simulink model "MultipleCoordinator"  (R2021b)
settings: Solver=FixedStepDiscrete  StartTime=0.0  StopTime=10.0  RelTol=1e-3
undefined symbols (not defined in the file): sldvsubsys
libraries: simulink x8, sldvlib x4
settings Model: Creator=Alessandro  LastModifiedBy=Mattia
settings ConfigComp: DVMode=PropertyProving  DVTestSuiteOptimization=Auto  DVDetectOutOfBounds=on  DVModelReferenceHarness=on

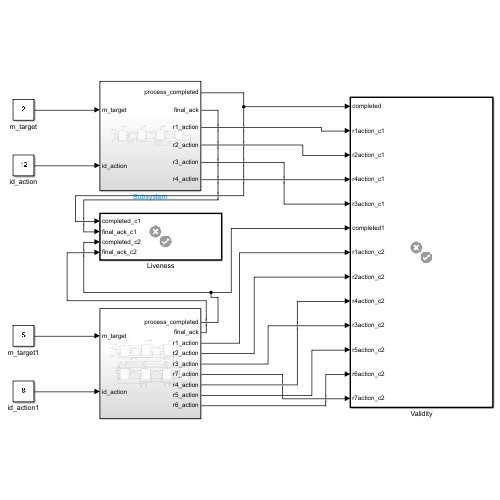
[thumbnail: Simulink's stored preview of the top-level diagram]
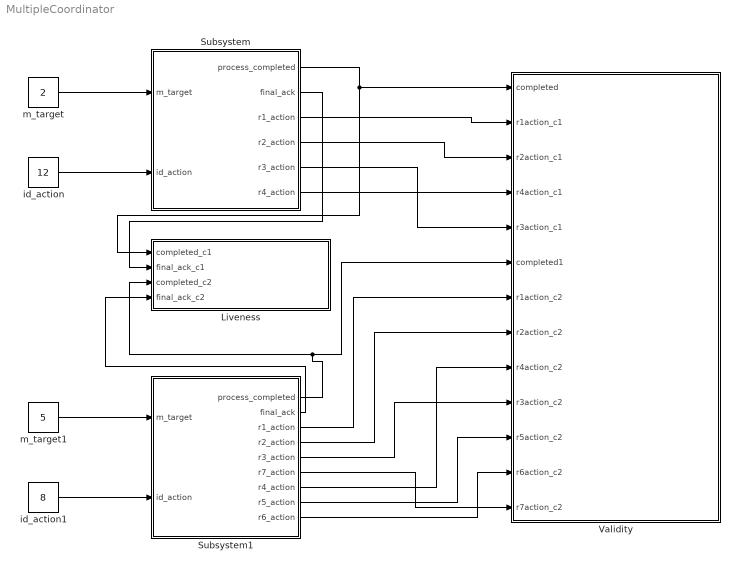
== system MultipleCoordinator ==
  Liveness : Subsystem  Tag=VerificationSubsystem  DisableCoverage=on  LoadFcn=sldvsubsys('check')  TreatAsAtomicUnit=on  SimViewingDevice=on  mask(VerificationSubsystem){}
      mask init:
      | sldvsubsys('maskInit');
      settings: CopyFcn=sldvsubsys('copy');  OpenFcn=open_system(gcb,'force');
      settings: PreSaveFcn=|
      | set_param(gcb,'SimViewingDevice','on');
      | sldvsubsys('check');
      mask Help: helpview(fullfile(docroot,'toolbox','sldv','sldv.map'),'verificationsubsystem')
      mask Display: image(imread('sldvicon_versubsys.png','BackGroundColor',[1 1 1]),'center');
  Subsystem : Subsystem
  Subsystem1 : Subsystem
  Validity : Subsystem  Tag=VerificationSubsystem  DisableCoverage=on  LoadFcn=sldvsubsys('check')  TreatAsAtomicUnit=on  SimViewingDevice=on  mask(VerificationSubsystem){}
      mask init:
      | sldvsubsys('maskInit');
      settings: CopyFcn=sldvsubsys('copy');  OpenFcn=open_system(gcb,'force');
      settings: PreSaveFcn=|
      | set_param(gcb,'SimViewingDevice','on');
      | sldvsubsys('check');
      mask Help: helpview(fullfile(docroot,'toolbox','sldv','sldv.map'),'verificationsubsystem')
      mask Display: image(imread('sldvicon_versubsys.png','BackGroundColor',[1 1 1]),'center');
  id_action : Constant  Value=12
  id_action1 : Constant  Value=8
  m_target : Constant  Value=2
  m_target1 : Constant  Value=5
  wires:
  m_target/1 -> Subsystem/1(m_target)
  id_action/1 -> Subsystem/2(id_action)
  Subsystem/1(process_completed) -> Liveness/1(completed_c1), Validity/1(completed)
  Subsystem/2(final_ack) -> Liveness/2(final_ack_c1)
  Subsystem/3(r1_action) -> Validity/2(r1action_c1)
  Subsystem/4(r2_action) -> Validity/3(r2action_c1)
  Subsystem/5(r3_action) -> Validity/5(r3action_c1)
  Subsystem/6(r4_action) -> Validity/4(r4action_c1)
  Subsystem1/2(final_ack) -> Liveness/4(final_ack_c2)
  id_action1/1 -> Subsystem1/2(id_action)
  m_target1/1 -> Subsystem1/1(m_target)
  Subsystem1/1(process_completed) -> Validity/6(completed1), Liveness/3(completed_c2)
  Subsystem1/3(r1_action) -> Validity/7(r1action_c2)
  Subsystem1/4(r2_action) -> Validity/8(r2action_c2)
  Subsystem1/7(r4_action) -> Validity/9(r4action_c2)
  Subsystem1/5(r3_action) -> Validity/10(r3action_c2)
  Subsystem1/8(r5_action) -> Validity/11(r5action_c2)
  Subsystem1/9(r6_action) -> Validity/12(r6action_c2)
  Subsystem1/6(r7_action) -> Validity/13(r7action_c2)

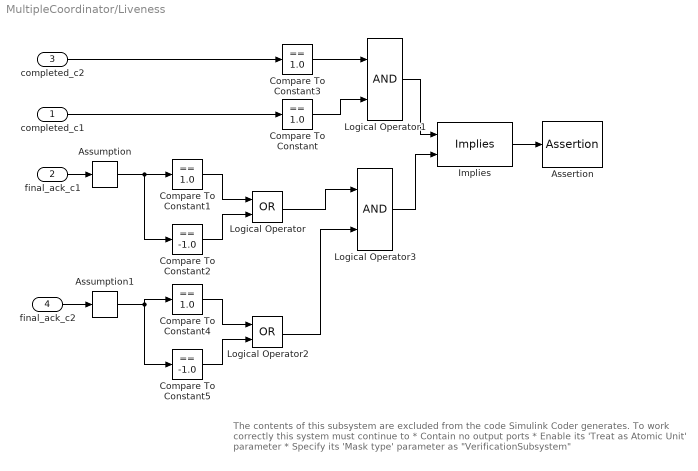
== system MultipleCoordinator/Liveness ==
  note: The contents of this subsystem are excluded from the code Simulink Coder
      | generates.
      |
      | To work correctly this system must continue to
      | * Contain no output ports
      | * Enable its 'Treat as Atomic Unit' parameter
      | * Specify its 'Mask type' parameter as "VerificationSubsystem"
  completed_c1 : Inport
  final_ack_c1 : Inport  Port=2
  completed_c2 : Inport  Port=3
  final_ack_c2 : Inport  Port=4
  Assertion : Assertion
  Assumption : sldvlib/Objectives and Constraints/Assumption  enabled=off  customAVTBlockType=Assumption  intervals={-1,1}  initial=off  dispValues=on  outEnabled=on
      settings: AttributesFormatString=%<intervals>  SourceProductBaseCode=SL
  Assumption1 : sldvlib/Objectives and Constraints/Assumption  enabled=off  customAVTBlockType=Assumption  intervals={-1,1}  initial=off  dispValues=on  outEnabled=on
      settings: AttributesFormatString=%<intervals>  SourceProductBaseCode=SL
  Compare To Constant{,1,3..4} (4 alike) : simulink/Logic and Bit Operations/Compare To Constant  relop===  const=1.0  OutDataTypeStr=boolean
  Compare To Constant2 : simulink/Logic and Bit Operations/Compare To Constant  relop===  const=-1.0  OutDataTypeStr=boolean
  Compare To Constant5 : simulink/Logic and Bit Operations/Compare To Constant  relop===  const=-1.0  OutDataTypeStr=boolean
  Implies : sldvlib/Verification Utilities/Implies
      settings: SourceProductBaseCode=SL
  Logical Operator : Logic  Operator=OR  AllPortsSameDT=off  OutDataTypeStr=boolean
  Logical Operator1 : Logic  AllPortsSameDT=off  OutDataTypeStr=boolean
  Logical Operator2 : Logic  Operator=OR  AllPortsSameDT=off  OutDataTypeStr=boolean
  Logical Operator3 : Logic  AllPortsSameDT=off  OutDataTypeStr=boolean
  wires:
  completed_c1/1 -> Compare To Constant/1
  Compare To Constant1/1 -> Logical Operator/1
  Compare To Constant2/1 -> Logical Operator/2
  Implies/1 -> Assertion/1
  final_ack_c1/1 -> Assumption/1
  Assumption/1 -> Compare To Constant2/1, Compare To Constant1/1
  completed_c2/1 -> Compare To Constant3/1
  Compare To Constant3/1 -> Logical Operator1/1
  Compare To Constant/1 -> Logical Operator1/2
  Compare To Constant4/1 -> Logical Operator2/1
  Compare To Constant5/1 -> Logical Operator2/2
  final_ack_c2/1 -> Assumption1/1
  Logical Operator1/1 -> Implies/1
  Logical Operator/1 -> Logical Operator3/1
  Logical Operator2/1 -> Logical Operator3/2
  Logical Operator3/1 -> Implies/2
  Assumption1/1 -> Compare To Constant4/1, Compare To Constant5/1

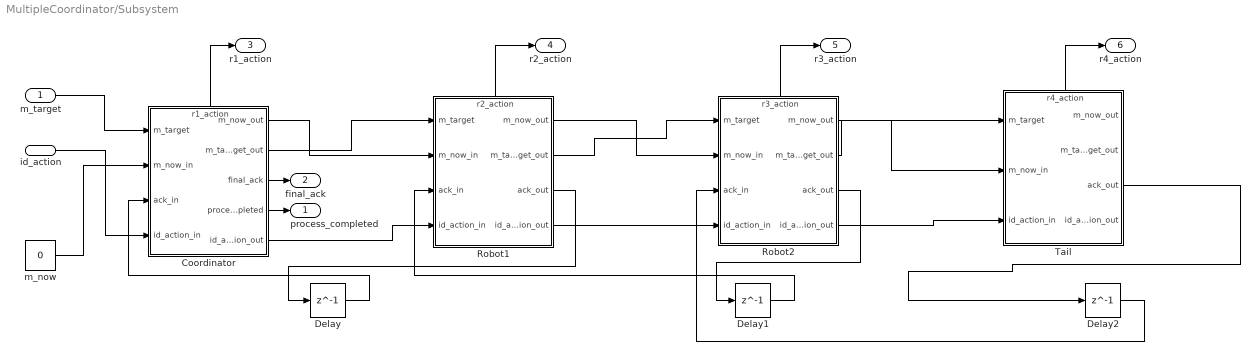
== system MultipleCoordinator/Subsystem ==
  m_target : Inport
  id_action : Inport  Port=2
  Coordinator : Stateflow chart  TreatAsAtomicUnit=on
      settings: PortSchema="{\"entries\":[{\"content\":{\"sides\":[{\"content\":{\"connectorIds\":[\"In1\",\"In2\",\"In3\",\"In4\"]},\"type\":\"ConnectorPlacement.EquallySpacedRectSide\",\"uuid\":\"f207236c-0599-4b46-9b3f-c0f809d9e1de\"},{\"content\":{\"connectorIds\":[\"Out2\",\"Out3\",\"Out4\",\"Out5\",\"Out6\"],\"side\":\"RIGHT\"},\"type\":\"ConnectorPlacement.EquallySpacedRectSide\",\"uuid\":\"63272974-e9ab-41b4-a3ca-cff66dd5b970\"},{\"content\":{\"connectorIds\":[\"Out1\"],\"side\":\"TOP\"},\"type\":\"ConnectorPlacement.EquallySpacedRectSide\",\"uuid\":\"6ce3df78-5d10-4d9a-bb6f-21eee9393606\"}]},\"type\":\"ConnectorPlacement.EquallySpacedConnector\",\"uuid\":\"1a0d068b-3bbf-4b25-a405-60ce12d31816\"}],\"packageUris\":[\"http://schema.mathworks.com/mf0/Connector/R2020b\"],\"version\":\"1.0\"}"
  Delay : Delay  DelayLength=1  InitialCondition=0
  Delay1 : Delay  DelayLength=1  InitialCondition=0
  Delay2 : Delay  DelayLength=1  InitialCondition=0
  Robot1 : Stateflow chart  TreatAsAtomicUnit=on
      settings: PortSchema="{\"entries\":[{\"content\":{\"sides\":[{\"content\":{\"connectorIds\":[\"In1\",\"In2\",\"In3\",\"In4\"]},\"type\":\"ConnectorPlacement.EquallySpacedRectSide\",\"uuid\":\"0bb30c5a-43df-4072-a77c-4a1dce14f9fe\"},{\"content\":{\"connectorIds\":[\"Out2\",\"Out3\",\"Out4\",\"Out5\"],\"side\":\"RIGHT\"},\"type\":\"ConnectorPlacement.EquallySpacedRectSide\",\"uuid\":\"e534c186-56c2-4af4-b3f1-02d020398bac\"},{\"content\":{\"connectorIds\":[\"Out1\"],\"side\":\"TOP\"},\"type\":\"ConnectorPlacement.EquallySpacedRectSide\",\"uuid\":\"e2ef603c-6980-4fc1-bc1c-88b0ffffdb44\"}]},\"type\":\"ConnectorPlacement.EquallySpacedConnector\",\"uuid\":\"7e88c6c9-7de7-4b98-93fa-510699497ff0\"}],\"packageUris\":[\"http://schema.mathworks.com/mf0/Connector/R2020b\"],\"version\":\"1.0\"}"
  Robot2 : Stateflow chart  TreatAsAtomicUnit=on
      settings: PortSchema="{\"entries\":[{\"content\":{\"sides\":[{\"content\":{\"connectorIds\":[\"In1\",\"In2\",\"In3\",\"In4\"]},\"type\":\"ConnectorPlacement.EquallySpacedRectSide\",\"uuid\":\"0bb30c5a-43df-4072-a77c-4a1dce14f9fe\"},{\"content\":{\"connectorIds\":[\"Out2\",\"Out3\",\"Out4\",\"Out5\"],\"side\":\"RIGHT\"},\"type\":\"ConnectorPlacement.EquallySpacedRectSide\",\"uuid\":\"e534c186-56c2-4af4-b3f1-02d020398bac\"},{\"content\":{\"connectorIds\":[\"Out1\"],\"side\":\"TOP\"},\"type\":\"ConnectorPlacement.EquallySpacedRectSide\",\"uuid\":\"e2ef603c-6980-4fc1-bc1c-88b0ffffdb44\"}]},\"type\":\"ConnectorPlacement.EquallySpacedConnector\",\"uuid\":\"7e88c6c9-7de7-4b98-93fa-510699497ff0\"}],\"packageUris\":[\"http://schema.mathworks.com/mf0/Connector/R2020b\"],\"version\":\"1.0\"}"
  Tail : Stateflow chart  TreatAsAtomicUnit=on
      settings: PortSchema="{\"entries\":[{\"content\":{\"sides\":[{\"content\":{\"connectorIds\":[\"In1\",\"In2\",\"In3\"]},\"type\":\"ConnectorPlacement.EquallySpacedRectSide\",\"uuid\":\"8f0c7a78-6297-425d-9fc8-91e71c821e74\"},{\"content\":{\"connectorIds\":[\"Out2\",\"Out3\",\"Out4\",\"Out5\"],\"side\":\"RIGHT\"},\"type\":\"ConnectorPlacement.EquallySpacedRectSide\",\"uuid\":\"2a4e4ba2-0ea2-4b66-9720-65f8c6802208\"},{\"content\":{\"connectorIds\":[\"Out1\"],\"side\":\"TOP\"},\"type\":\"ConnectorPlacement.EquallySpacedRectSide\",\"uuid\":\"3c4e4337-d1ab-4209-abe4-e09ccc9a45b1\"}]},\"type\":\"ConnectorPlacement.EquallySpacedConnector\",\"uuid\":\"5f75d573-6dad-4549-ba0d-242a5d54a9e5\"}],\"packageUris\":[\"http://schema.mathworks.com/mf0/Connector/R2020b\"],\"version\":\"1.0\"}"
  m_now : Constant  Value=0
  process_completed : Outport
  final_ack : Outport  Port=2
  r1_action : Outport  Port=3
  r2_action : Outport  Port=4
  r3_action : Outport  Port=5
  r4_action : Outport  Port=6
  wires:
  m_now/1 -> Coordinator/2(m_now_in)
  m_target/1 -> Coordinator/1(m_target)
  Delay/1 -> Coordinator/3(ack_in)
  Coordinator/2(m_now_out) -> Robot1/2(m_now_in)
  Coordinator/3(m_target_out) -> Robot1/1(m_target)
  Robot1/4(ack_out) -> Delay/1
  Coordinator/5(process_completed) -> process_completed/1
  Coordinator/4(final_ack) -> final_ack/1
  id_action/1 -> Coordinator/4(id_action_in)
  Coordinator/6(id_action_out) -> Robot1/4(id_action_in)
  Robot1/2(m_now_out) -> Robot2/2(m_now_in)
  Robot1/3(m_target_out) -> Robot2/1(m_target)
  Robot1/5(id_action_out) -> Robot2/4(id_action_in)
  Robot2/2(m_now_out) -> Tail/2(m_now_in)
  Robot2/3(m_target_out) -> Tail/1(m_target)
  Robot2/5(id_action_out) -> Tail/3(id_action_in)
  Robot2/4(ack_out) -> Delay1/1
  Delay1/1 -> Robot1/3(ack_in)
  Tail/4(ack_out) -> Delay2/1
  Delay2/1 -> Robot2/3(ack_in)
  Coordinator/1(r1_action) -> r1_action/1
  Robot1/1(r2_action) -> r2_action/1
  Robot2/1(r3_action) -> r3_action/1
  Tail/1(r4_action) -> r4_action/1

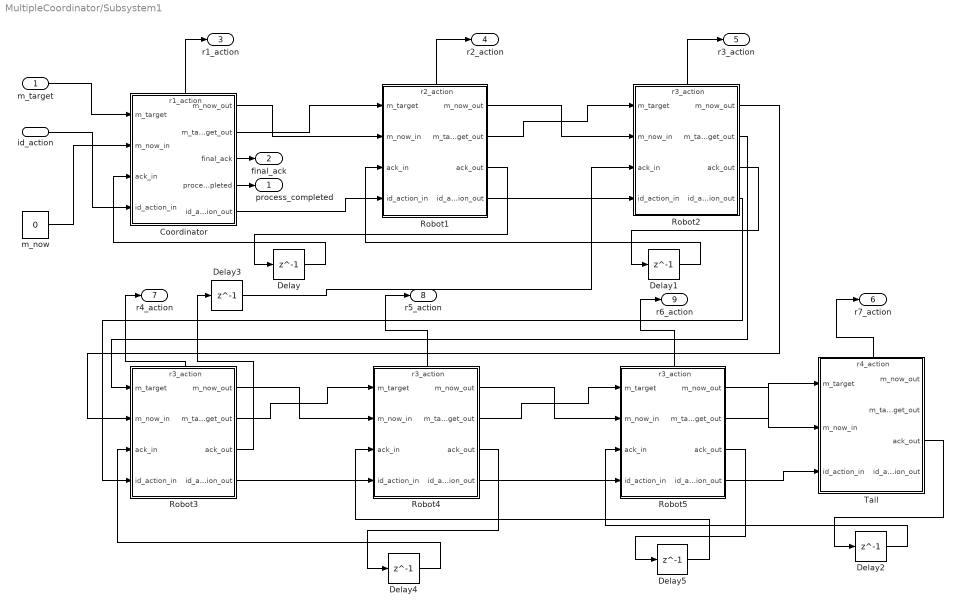
== system MultipleCoordinator/Subsystem1 ==
  m_target : Inport
  id_action : Inport  Port=2
  Coordinator : Stateflow chart  TreatAsAtomicUnit=on
      settings: PortSchema="{\"entries\":[{\"content\":{\"sides\":[{\"content\":{\"connectorIds\":[\"In1\",\"In2\",\"In3\",\"In4\"]},\"type\":\"ConnectorPlacement.EquallySpacedRectSide\",\"uuid\":\"f207236c-0599-4b46-9b3f-c0f809d9e1de\"},{\"content\":{\"connectorIds\":[\"Out2\",\"Out3\",\"Out4\",\"Out5\",\"Out6\"],\"side\":\"RIGHT\"},\"type\":\"ConnectorPlacement.EquallySpacedRectSide\",\"uuid\":\"63272974-e9ab-41b4-a3ca-cff66dd5b970\"},{\"content\":{\"connectorIds\":[\"Out1\"],\"side\":\"TOP\"},\"type\":\"ConnectorPlacement.EquallySpacedRectSide\",\"uuid\":\"6ce3df78-5d10-4d9a-bb6f-21eee9393606\"}]},\"type\":\"ConnectorPlacement.EquallySpacedConnector\",\"uuid\":\"1a0d068b-3bbf-4b25-a405-60ce12d31816\"}],\"packageUris\":[\"http://schema.mathworks.com/mf0/Connector/R2020b\"],\"version\":\"1.0\"}"
  Delay{,1..5} (6 alike) : Delay  DelayLength=1  InitialCondition=0
  Robot1 : Stateflow chart  TreatAsAtomicUnit=on
      settings: PortSchema="{\"entries\":[{\"content\":{\"sides\":[{\"content\":{\"connectorIds\":[\"In1\",\"In2\",\"In3\",\"In4\"]},\"type\":\"ConnectorPlacement.EquallySpacedRectSide\",\"uuid\":\"0bb30c5a-43df-4072-a77c-4a1dce14f9fe\"},{\"content\":{\"connectorIds\":[\"Out2\",\"Out3\",\"Out4\",\"Out5\"],\"side\":\"RIGHT\"},\"type\":\"ConnectorPlacement.EquallySpacedRectSide\",\"uuid\":\"e534c186-56c2-4af4-b3f1-02d020398bac\"},{\"content\":{\"connectorIds\":[\"Out1\"],\"side\":\"TOP\"},\"type\":\"ConnectorPlacement.EquallySpacedRectSide\",\"uuid\":\"e2ef603c-6980-4fc1-bc1c-88b0ffffdb44\"}]},\"type\":\"ConnectorPlacement.EquallySpacedConnector\",\"uuid\":\"7e88c6c9-7de7-4b98-93fa-510699497ff0\"}],\"packageUris\":[\"http://schema.mathworks.com/mf0/Connector/R2020b\"],\"version\":\"1.0\"}"
  Robot2 : Stateflow chart  TreatAsAtomicUnit=on
      settings: PortSchema="{\"entries\":[{\"content\":{\"sides\":[{\"content\":{\"connectorIds\":[\"In1\",\"In2\",\"In3\",\"In4\"]},\"type\":\"ConnectorPlacement.EquallySpacedRectSide\",\"uuid\":\"0bb30c5a-43df-4072-a77c-4a1dce14f9fe\"},{\"content\":{\"connectorIds\":[\"Out2\",\"Out3\",\"Out4\",\"Out5\"],\"side\":\"RIGHT\"},\"type\":\"ConnectorPlacement.EquallySpacedRectSide\",\"uuid\":\"e534c186-56c2-4af4-b3f1-02d020398bac\"},{\"content\":{\"connectorIds\":[\"Out1\"],\"side\":\"TOP\"},\"type\":\"ConnectorPlacement.EquallySpacedRectSide\",\"uuid\":\"e2ef603c-6980-4fc1-bc1c-88b0ffffdb44\"}]},\"type\":\"ConnectorPlacement.EquallySpacedConnector\",\"uuid\":\"7e88c6c9-7de7-4b98-93fa-510699497ff0\"}],\"packageUris\":[\"http://schema.mathworks.com/mf0/Connector/R2020b\"],\"version\":\"1.0\"}"
  Robot3 : Stateflow chart  TreatAsAtomicUnit=on
      settings: PortSchema="{\"entries\":[{\"content\":{\"sides\":[{\"content\":{\"connectorIds\":[\"In1\",\"In2\",\"In3\",\"In4\"]},\"type\":\"ConnectorPlacement.EquallySpacedRectSide\",\"uuid\":\"0bb30c5a-43df-4072-a77c-4a1dce14f9fe\"},{\"content\":{\"connectorIds\":[\"Out2\",\"Out3\",\"Out4\",\"Out5\"],\"side\":\"RIGHT\"},\"type\":\"ConnectorPlacement.EquallySpacedRectSide\",\"uuid\":\"e534c186-56c2-4af4-b3f1-02d020398bac\"},{\"content\":{\"connectorIds\":[\"Out1\"],\"side\":\"TOP\"},\"type\":\"ConnectorPlacement.EquallySpacedRectSide\",\"uuid\":\"e2ef603c-6980-4fc1-bc1c-88b0ffffdb44\"}]},\"type\":\"ConnectorPlacement.EquallySpacedConnector\",\"uuid\":\"7e88c6c9-7de7-4b98-93fa-510699497ff0\"}],\"packageUris\":[\"http://schema.mathworks.com/mf0/Connector/R2020b\"],\"version\":\"1.0\"}"
  Robot4 : Stateflow chart  TreatAsAtomicUnit=on
      settings: PortSchema="{\"entries\":[{\"content\":{\"sides\":[{\"content\":{\"connectorIds\":[\"In1\",\"In2\",\"In3\",\"In4\"]},\"type\":\"ConnectorPlacement.EquallySpacedRectSide\",\"uuid\":\"0bb30c5a-43df-4072-a77c-4a1dce14f9fe\"},{\"content\":{\"connectorIds\":[\"Out2\",\"Out3\",\"Out4\",\"Out5\"],\"side\":\"RIGHT\"},\"type\":\"ConnectorPlacement.EquallySpacedRectSide\",\"uuid\":\"e534c186-56c2-4af4-b3f1-02d020398bac\"},{\"content\":{\"connectorIds\":[\"Out1\"],\"side\":\"TOP\"},\"type\":\"ConnectorPlacement.EquallySpacedRectSide\",\"uuid\":\"e2ef603c-6980-4fc1-bc1c-88b0ffffdb44\"}]},\"type\":\"ConnectorPlacement.EquallySpacedConnector\",\"uuid\":\"7e88c6c9-7de7-4b98-93fa-510699497ff0\"}],\"packageUris\":[\"http://schema.mathworks.com/mf0/Connector/R2020b\"],\"version\":\"1.0\"}"
  Robot5 : Stateflow chart  TreatAsAtomicUnit=on
      settings: PortSchema="{\"entries\":[{\"content\":{\"sides\":[{\"content\":{\"connectorIds\":[\"In1\",\"In2\",\"In3\",\"In4\"]},\"type\":\"ConnectorPlacement.EquallySpacedRectSide\",\"uuid\":\"0bb30c5a-43df-4072-a77c-4a1dce14f9fe\"},{\"content\":{\"connectorIds\":[\"Out2\",\"Out3\",\"Out4\",\"Out5\"],\"side\":\"RIGHT\"},\"type\":\"ConnectorPlacement.EquallySpacedRectSide\",\"uuid\":\"e534c186-56c2-4af4-b3f1-02d020398bac\"},{\"content\":{\"connectorIds\":[\"Out1\"],\"side\":\"TOP\"},\"type\":\"ConnectorPlacement.EquallySpacedRectSide\",\"uuid\":\"e2ef603c-6980-4fc1-bc1c-88b0ffffdb44\"}]},\"type\":\"ConnectorPlacement.EquallySpacedConnector\",\"uuid\":\"7e88c6c9-7de7-4b98-93fa-510699497ff0\"}],\"packageUris\":[\"http://schema.mathworks.com/mf0/Connector/R2020b\"],\"version\":\"1.0\"}"
  Tail : Stateflow chart  TreatAsAtomicUnit=on
      settings: PortSchema="{\"entries\":[{\"content\":{\"sides\":[{\"content\":{\"connectorIds\":[\"In1\",\"In2\",\"In3\"]},\"type\":\"ConnectorPlacement.EquallySpacedRectSide\",\"uuid\":\"8f0c7a78-6297-425d-9fc8-91e71c821e74\"},{\"content\":{\"connectorIds\":[\"Out2\",\"Out3\",\"Out4\",\"Out5\"],\"side\":\"RIGHT\"},\"type\":\"ConnectorPlacement.EquallySpacedRectSide\",\"uuid\":\"2a4e4ba2-0ea2-4b66-9720-65f8c6802208\"},{\"content\":{\"connectorIds\":[\"Out1\"],\"side\":\"TOP\"},\"type\":\"ConnectorPlacement.EquallySpacedRectSide\",\"uuid\":\"3c4e4337-d1ab-4209-abe4-e09ccc9a45b1\"}]},\"type\":\"ConnectorPlacement.EquallySpacedConnector\",\"uuid\":\"5f75d573-6dad-4549-ba0d-242a5d54a9e5\"}],\"packageUris\":[\"http://schema.mathworks.com/mf0/Connector/R2020b\"],\"version\":\"1.0\"}"
  m_now : Constant  Value=0
  process_completed : Outport
  final_ack : Outport  Port=2
  r1_action : Outport  Port=3
  r2_action : Outport  Port=4
  r3_action : Outport  Port=5
  r7_action : Outport  Port=6
  r4_action : Outport  Port=7
  r5_action : Outport  Port=8
  r6_action : Outport  Port=9
  wires:
  m_now/1 -> Coordinator/2(m_now_in)
  m_target/1 -> Coordinator/1(m_target)
  Delay/1 -> Coordinator/3(ack_in)
  Coordinator/2(m_now_out) -> Robot1/2(m_now_in)
  Coordinator/3(m_target_out) -> Robot1/1(m_target)
  Robot1/4(ack_out) -> Delay/1
  Coordinator/5(process_completed) -> process_completed/1
  Coordinator/4(final_ack) -> final_ack/1
  id_action/1 -> Coordinator/4(id_action_in)
  Coordinator/6(id_action_out) -> Robot1/4(id_action_in)
  Robot1/2(m_now_out) -> Robot2/2(m_now_in)
  Robot1/3(m_target_out) -> Robot2/1(m_target)
  Robot1/5(id_action_out) -> Robot2/4(id_action_in)
  Robot2/4(ack_out) -> Delay1/1
  Delay1/1 -> Robot1/3(ack_in)
  Tail/4(ack_out) -> Delay2/1
  Coordinator/1(r1_action) -> r1_action/1
  Robot1/1(r2_action) -> r2_action/1
  Robot2/1(r3_action) -> r3_action/1
  Tail/1(r4_action) -> r7_action/1
  Robot2/3(m_target_out) -> Robot3/1(m_target)
  Robot3/1(r3_action) -> r4_action/1
  Delay3/1 -> Robot2/3(ack_in)
  Robot3/4(ack_out) -> Delay3/1
  Robot2/5(id_action_out) -> Robot3/4(id_action_in)
  Robot2/2(m_now_out) -> Robot3/2(m_now_in)
  Robot3/3(m_target_out) -> Robot4/1(m_target)
  Robot4/1(r3_action) -> r5_action/1
  Delay4/1 -> Robot3/3(ack_in)
  Robot4/4(ack_out) -> Delay4/1
  Robot3/5(id_action_out) -> Robot4/4(id_action_in)
  Robot3/2(m_now_out) -> Robot4/2(m_now_in)
  Robot4/3(m_target_out) -> Robot5/1(m_target)
  Robot5/1(r3_action) -> r6_action/1
  Delay5/1 -> Robot4/3(ack_in)
  Robot5/4(ack_out) -> Delay5/1
  Robot4/5(id_action_out) -> Robot5/4(id_action_in)
  Robot4/2(m_now_out) -> Robot5/2(m_now_in)
  Robot5/3(m_target_out) -> Tail/1(m_target)
  Robot5/2(m_now_out) -> Tail/2(m_now_in)
  Delay2/1 -> Robot5/3(ack_in)
  Robot5/5(id_action_out) -> Tail/3(id_action_in)

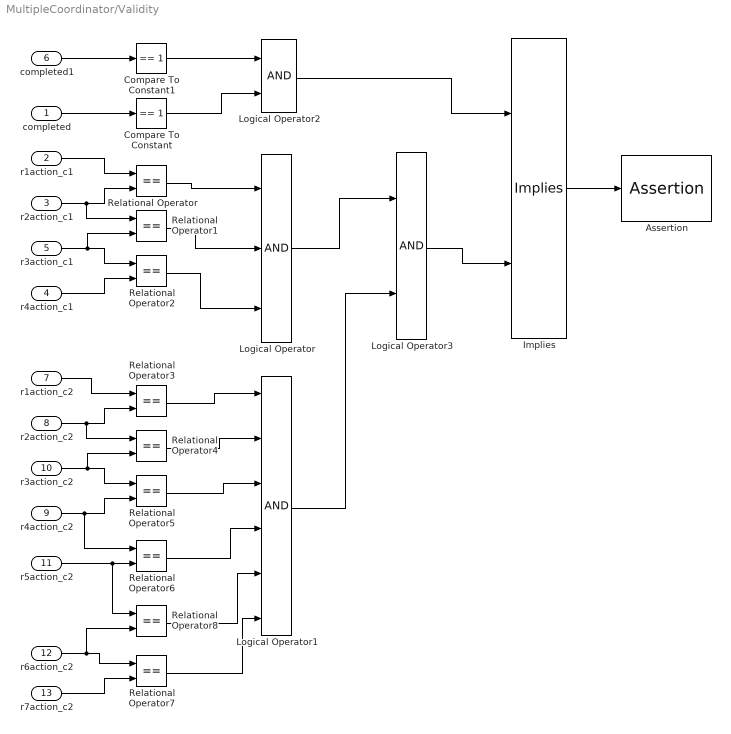
== system MultipleCoordinator/Validity ==
  completed : Inport
  r1action_c1 : Inport  Port=2
  r2action_c1 : Inport  Port=3
  r4action_c1 : Inport  Port=4
  r3action_c1 : Inport  Port=5
  completed1 : Inport  Port=6
  r1action_c2 : Inport  Port=7
  r2action_c2 : Inport  Port=8
  r4action_c2 : Inport  Port=9
  r3action_c2 : Inport  Port=10
  r5action_c2 : Inport  Port=11
  r6action_c2 : Inport  Port=12
  r7action_c2 : Inport  Port=13
  Assertion : Assertion
  Compare To Constant : simulink/Logic and Bit Operations/Compare To Constant  relop===  const=1  OutDataTypeStr=boolean
  Compare To Constant1 : simulink/Logic and Bit Operations/Compare To Constant  relop===  const=1  OutDataTypeStr=boolean
  Implies : sldvlib/Verification Utilities/Implies
      settings: SourceProductBaseCode=SL
  Logical Operator : Logic  Inputs=3  AllPortsSameDT=off  OutDataTypeStr=boolean
  Logical Operator1 : Logic  Inputs=6  AllPortsSameDT=off  OutDataTypeStr=boolean
  Logical Operator2 : Logic  AllPortsSameDT=off  OutDataTypeStr=boolean
  Logical Operator3 : Logic  AllPortsSameDT=off  OutDataTypeStr=boolean
  Relational Operator{,1..8} (9 alike) : RelationalOperator  Operator===  OutDataTypeStr=boolean  RndMeth=Simplest
  wires:
  completed/1 -> Compare To Constant/1
  Relational Operator/1 -> Logical Operator/1
  Relational Operator1/1 -> Logical Operator/2
  Relational Operator2/1 -> Logical Operator/3
  r1action_c1/1 -> Relational Operator/1
  r2action_c1/1 -> Relational Operator1/1, Relational Operator/2
  r3action_c1/1 -> Relational Operator1/2, Relational Operator2/1
  r4action_c1/1 -> Relational Operator2/2
  r2action_c2/1 -> Relational Operator4/1, Relational Operator3/2
  Relational Operator4/1 -> Logical Operator1/2
  r7action_c2/1 -> Relational Operator7/2
  r4action_c2/1 -> Relational Operator6/1, Relational Operator5/2
  r1action_c2/1 -> Relational Operator3/1
  r5action_c2/1 -> Relational Operator8/1, Relational Operator6/2
  r6action_c2/1 -> Relational Operator8/2, Relational Operator7/1
  Relational Operator6/1 -> Logical Operator1/4
  Relational Operator8/1 -> Logical Operator1/5
  r3action_c2/1 -> Relational Operator4/2, Relational Operator5/1
  Relational Operator5/1 -> Logical Operator1/3
  Relational Operator3/1 -> Logical Operator1/1
  completed1/1 -> Compare To Constant1/1
  Relational Operator7/1 -> Logical Operator1/6
  Compare To Constant1/1 -> Logical Operator2/1
  Compare To Constant/1 -> Logical Operator2/2
  Logical Operator/1 -> Logical Operator3/1
  Logical Operator1/1 -> Logical Operator3/2
  Implies/1 -> Assertion/1
  Logical Operator2/1 -> Implies/1
  Logical Operator3/1 -> Implies/2

== stateflow chart MultipleCoordinator/Subsystem1/Coordinator ==
  state FeedForward
    entry:
    m_target_out = m_target
    id_action_out = id_action_in;
  state Initial
    entry:
    r1_action = id_action_in;
    gen = Random();
    if gen>0.5
    m_now_out = m_now_in + 1;
    end
  state EnoughRobots1
    process_completed=1;
    final_ack = ack_in;
  (default) -> Initial
  Initial -> FeedForward
  FeedForward -> EnoughRobots1 : [ack_in == 1 || ack_in == -1]
  data: r function_output; r1_action output; m_target input; m_now_in input; m_now_out output; gen local; m_target_out output; ack_in input; final_ack output; process_completed output; id_action_in input; id_action_out output
  function r = Random:
    | function r = Random
    | %#codegen
    | rng(1);
    | r = rand(1);
    | end

== stateflow chart MultipleCoordinator/Subsystem1/Robot1 ==
  state FeedForward
    entry:
    r2_action = id_action_in;
    m_target_out = m_target
    id_action_out = id_action_in;
  state Initial
    entry:
    gen = 0;
    if gen>0.5
    m_now_out = m_now_in + 1;
    end
  state EnoughRobots1
    entry:
    r2_action = id_action_in;
    ack_out = ack_in;
  (default) -> Initial
  Initial -> FeedForward
  FeedForward -> EnoughRobots1 : [ack_in == 1 || ack_in == -1]
  data: r function_output; r2_action output; m_target input; m_now_in input; m_now_out output; gen local; m_target_out output; ack_in input; ack_out output; id_action_in input; id_action_out output
  function r = Random:
    | function r = Random
    | %#codegen
    | rng(2);
    | r = rand(1);
    | end

== stateflow chart MultipleCoordinator/Subsystem1/Robot2 ==
  state FeedForward
    entry:
    m_target_out = m_target
    id_action_out = id_action_in;
    r3_action = id_action_in;
  state Initial
    entry:
    r3_action = id_action_in;
    gen = 0;
    if gen>0.5
    m_now_out = m_now_in + 1;
    end
  state EnoughRobots1
    entry:
    ack_out = ack_in;
    r3_action = id_action_in;
  (default) -> Initial
  Initial -> FeedForward
  FeedForward -> EnoughRobots1 : [ack_in == 1 || ack_in == -1]
  data: r function_output; r3_action output; m_target input; m_now_in input; m_now_out output; gen local; m_target_out output; ack_in input; ack_out output; id_action_in input; id_action_out output
  function r = Random:
    | function r = Random
    | %#codegen
    | rng(3);
    | r = rand(1);
    | end

== stateflow chart MultipleCoordinator/Subsystem1/Robot3 ==
  state FeedForward
    entry:
    m_target_out = m_target
    id_action_out = id_action_in;
    r3_action = id_action_in;
  state Initial
    entry:
    r3_action = id_action_in;
    gen = Random();
    if gen>0.5
    m_now_out = m_now_in + 1;
    end
  state EnoughRobots1
    entry:
    ack_out = ack_in;
    r3_action = id_action_in;
  (default) -> Initial
  Initial -> FeedForward
  FeedForward -> EnoughRobots1 : [ack_in == 1 || ack_in == -1]
  data: r function_output; r3_action output; m_target input; m_now_in input; m_now_out output; gen local; m_target_out output; ack_in input; ack_out output; id_action_in input; id_action_out output
  function r = Random:
    | function r = Random
    | %#codegen
    | rng(3);
    | r = rand(1);
    | end

== stateflow chart MultipleCoordinator/Subsystem1/Robot4 ==
  state FeedForward
    entry:
    m_target_out = m_target
    id_action_out = id_action_in;
    r3_action = id_action_in;
  state Initial
    entry:
    r3_action = id_action_in;
    gen = 0;
    if gen>0.5
    m_now_out = m_now_in + 1;
    end
  state EnoughRobots1
    entry:
    ack_out = ack_in;
    r3_action = id_action_in;
  (default) -> Initial
  Initial -> FeedForward
  FeedForward -> EnoughRobots1 : [ack_in == 1 || ack_in == -1]
  data: r function_output; r3_action output; m_target input; m_now_in input; m_now_out output; gen local; m_target_out output; ack_in input; ack_out output; id_action_in input; id_action_out output
  function r = Random:
    | function r = Random
    | %#codegen
    | rng(3);
    | r = rand(1);
    | end

== stateflow chart MultipleCoordinator/Subsystem1/Robot5 ==
  state FeedForward
    entry:
    m_target_out = m_target
    id_action_out = id_action_in;
    r3_action = id_action_in;
  state Initial
    entry:
    r3_action = id_action_in;
    gen = Random();
    if gen>0.5
    m_now_out = m_now_in + 1;
    end
  state EnoughRobots1
    entry:
    ack_out = ack_in;
    r3_action = id_action_in;
  (default) -> Initial
  Initial -> FeedForward
  FeedForward -> EnoughRobots1 : [ack_in == 1 || ack_in == -1]
  data: r function_output; r3_action output; m_target input; m_now_in input; m_now_out output; gen local; m_target_out output; ack_in input; ack_out output; id_action_in input; id_action_out output
  function r = Random:
    | function r = Random
    | %#codegen
    | rng(3);
    | r = rand(1);
    | end

== stateflow chart MultipleCoordinator/Subsystem1/Tail ==
  state FeedForward
    entry:
    ack_out  = 1;
    r4_action = id_action_in;
  state Initial
    entry:
    r4_action = id_action_in;
    id_action_out = id_action_in;
    gen = 0;
    if gen>0.5
    m_now_out = m_now_in + 1;
    else
    m_now_out = m_now_in;
    end
  state EnoughRobots
    entry:
    ack_out  = -1;
    r4_action = id_action_in;
    m_target_out = m_target;
  (default) -> Initial
  Initial -> FeedForward [order 2] : [m_now_out >= m_target]
  Initial -> EnoughRobots [order 1] : [m_now_out < m_target]
  data: r function_output; r4_action output; m_target input; m_now_in input; m_now_out output; gen local; m_target_out output; ack_out output; id_action_in input; id_action_out output
  function r = Random:
    | function r = Random
    | %#codegen
    | rng(4);
    | r = rand(1);
    | end

== stateflow chart MultipleCoordinator/Subsystem/Robot1 ==
  state FeedForward
    entry:
    r2_action = id_action_in;
    m_target_out = m_target
    id_action_out = id_action_in;
  state Initial
    entry:
    gen = 0;
    if gen>0.5
    m_now_out = m_now_in + 1;
    end
  state EnoughRobots1
    entry:
    r2_action = id_action_in;
    ack_out = ack_in;
  (default) -> Initial
  Initial -> FeedForward
  FeedForward -> EnoughRobots1 : [ack_in == 1 || ack_in == -1]
  data: r function_output; r2_action output; m_target input; m_now_in input; m_now_out output; gen local; m_target_out output; ack_in input; ack_out output; id_action_in input; id_action_out output
  function r = Random:
    | function r = Random
    | %#codegen
    | rng(2);
    | r = rand(1);
    | end

== stateflow chart MultipleCoordinator/Subsystem/Tail ==
  state FeedForward
    entry:
    ack_out  = 1;
    r4_action = id_action_in;
  state Initial
    entry:
    r4_action = id_action_in;
    id_action_out = id_action_in;
    gen = Random();
    if gen>0.5
    m_now_out = m_now_in + 1;
    else
    m_now_out = m_now_in;
    end
  state EnoughRobots
    entry:
    ack_out  = -1;
    r4_action = id_action_in;
    m_target_out = m_target;
  (default) -> Initial
  Initial -> FeedForward [order 2] : [m_now_out >= m_target]
  Initial -> EnoughRobots [order 1] : [m_now_out < m_target]
  data: r function_output; r4_action output; m_target input; m_now_in input; m_now_out output; gen local; m_target_out output; ack_out output; id_action_in input; id_action_out output
  function r = Random:
    | function r = Random
    | %#codegen
    | rng(4);
    | r = rand(1);
    | end

== stateflow chart MultipleCoordinator/Subsystem/Coordinator ==
  state FeedForward
    entry:
    m_target_out = m_target
    id_action_out = id_action_in;
  state Initial
    entry:
    r1_action = id_action_in;
    gen = Random();
    if gen>0.5
    m_now_out = m_now_in + 1;
    end
  state EnoughRobots1
    process_completed=1;
    final_ack = ack_in;
  (default) -> Initial
  Initial -> FeedForward
  FeedForward -> EnoughRobots1 : [ack_in == 1 || ack_in == -1]
  data: r function_output; r1_action output; m_target input; m_now_in input; m_now_out output; gen local; m_target_out output; ack_in input; final_ack output; process_completed output; id_action_in input; id_action_out output
  function r = Random:
    | function r = Random
    | %#codegen
    | rng(1);
    | r = rand(1);
    | end

== stateflow chart MultipleCoordinator/Subsystem/Robot2 ==
  state FeedForward
    entry:
    m_target_out = m_target
    id_action_out = id_action_in;
    r3_action = id_action_in;
  state Initial
    entry:
    r3_action = id_action_in;
    gen = 0;
    if gen>0.5
    m_now_out = m_now_in + 1;
    end
  state EnoughRobots1
    entry:
    ack_out = ack_in;
    r3_action = id_action_in;
  (default) -> Initial
  Initial -> FeedForward
  FeedForward -> EnoughRobots1 : [ack_in == 1 || ack_in == -1]
  data: r function_output; r3_action output; m_target input; m_now_in input; m_now_out output; gen local; m_target_out output; ack_in input; ack_out output; id_action_in input; id_action_out output
  function r = Random:
    | function r = Random
    | %#codegen
    | rng(3);
    | r = rand(1);
    | end
